simulink model "exercise_3_2"  (R2017a)
settings: Solver=FixedStepAuto  StartTime=0.0  StopTime=simTime  FixedStep=Ts  RelTol=1e-3
values from neighbouring files (symbols this model uses):
  Disturbance = 1    [exercise_3.m]
  stepTime = 1    [exercise_3.m]
libraries: cstblocks x2
settings Model: Creator=marce  LastModifiedBy=marce

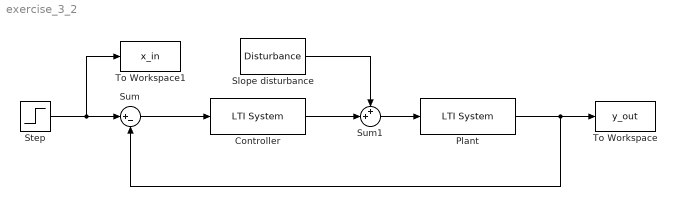
== system exercise_3_2 ==
  Controller : cstblocks/LTI System  sys=C  IC=[]
  Plant : cstblocks/LTI System  sys=H  IC=[]
  Slope disturbance : Constant  Value=Disturbance
  Step : Step  Time=stepTime  SampleTime=0
  Sum : Sum  Inputs=|+-
  Sum1 : Sum  Inputs=++|
  To Workspace : ToWorkspace  VariableName=y_out  SaveFormat=Timeseries  SampleTime=-1
  To Workspace1 : ToWorkspace  VariableName=x_in  SaveFormat=Timeseries  SampleTime=-1
  wires:
  Step/1 -> To Workspace1/1, Sum/1
  Plant/1 -> Sum/2, To Workspace/1
  Sum/1 -> Controller/1
  Slope disturbance/1 -> Sum1/1
  Sum1/1 -> Plant/1
  Controller/1 -> Sum1/2
